simulink model "sf_bounce"  (Simulink 7.6)
settings: Solver=ode15s  StartTime=0.0  StopTime=10  MaxStep=.1  RelTol=1e-6
settings Model: Creator=The MathWorks Inc.  ExtModeAutoUpdateStatusClock=off
settings SolverCC: ConsecutiveZCsStepRelTol=1*128*eps  ZeroCrossControl=EnableAll
settings DataIOCC: LimitDataPoints=off  SaveFormat=StructureWithTime
settings OptimizationCC: InitFltsAndDblsToZero=on  EfficientMapNaN2IntZero=off
settings DebuggingCC: SignalResolutionControl=TryResolveAllWithWarning  StrictBusMsg=Warning
settings HardwareCC: TargetEndianess=LittleEndian  TargetHWDeviceType=MATLAB Host
settings SFSimCC: SFSimEnableDebug=off  SFSimOverflowDetection=off  SFSimEcho=off  SimParseCustomCode=off
settings RTWCC: ProcessScript=grt_make_rtw_hook

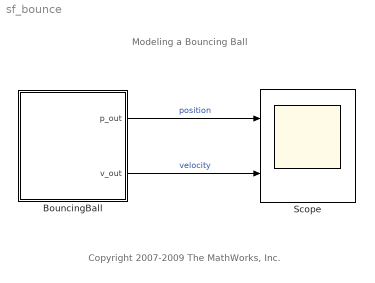
== system sf_bounce ==
  note: Modeling a Bouncing Ball
  note: Copyright 2007-2009 The MathWorks, Inc.
  BouncingBall : Stateflow chart  TreatAsAtomicUnit=on
  Scope : Scope  NumInputPorts=2
      settings: YMin=0~-30  YMax=25~20
  wires:
  BouncingBall/1(p_out) -> Scope/1  "position"
  BouncingBall/2(v_out) -> Scope/2  "velocity"

== stateflow chart BouncingBall ==
  settings: updateMethod=CONTINUOUS  executeAtInitialization=1  initializeOutput=1
  state Falling
    du:
    // derivatives
    p_dot = v;
    v_dot = -9.81;
    // outputs
    p_out = p;
    v_out = v;
  Falling -> Falling : [ p <= 0  && v < 0 ]
      | {
      | p = 0;
      | v = -0.8*v;
      | }
  (default) -> Falling : {
      | p = 10;
      | v = 15;
      | }
  data: p_out output double size=1; p local double =3; v local double; v_out output double size=1
  data p settings: updateMethod=SF_CONTINUOUS_TIME_DATA
  data v settings: updateMethod=SF_CONTINUOUS_TIME_DATA
